simulink model "ev_battery"  (Simulink 8.1)
settings: Solver=ode3  StartTime=0  StopTime=7579  FixedStep=1  RelTol=1e-3
libraries: CampusEnergyModeling x1
settings Model: Creator=sfrank1  LastModifiedBy=sfrank1
settings DataIOCC: SignalLoggingSaveFormat=Dataset
settings OptimizationCC: ExpressionDepthLimit=128
settings DebuggingCC: FcnCallInpInsideContextMsg=EnableAllAsError
settings GRTTargetCC: CombineOutputUpdateFcns=on  GRTInterface=off

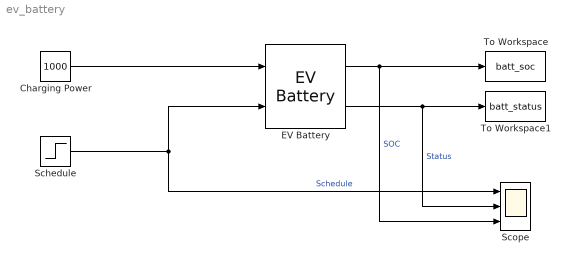
== system ev_battery ==
  Charging Power : Constant  Value=1000
  EV Battery : CampusEnergyModeling/Electric Vehicles/EV Battery  capacity=1000  initSOC=0  eff=0.95
  Schedule : Step  Time=1895  SampleTime=0
  Scope : Scope  NumInputPorts=3
      settings: YMin=-5~-5~-5  YMax=5~5~5
  To Workspace : ToWorkspace  VariableName=batt_soc  SampleTime=-1  SaveFormat=Timeseries
  To Workspace1 : ToWorkspace  VariableName=batt_status  SampleTime=-1  SaveFormat=Timeseries
  wires:
  Charging Power/1 -> EV Battery/1
  Schedule/1 -> Scope/1, EV Battery/2  "Schedule"
  EV Battery/1 -> Scope/3, To Workspace/1  "SOC"
  EV Battery/2 -> Scope/2, To Workspace1/1  "Status"
